simulink model "pe_pmsm_drive_code"  (R2018b)
settings: Solver=FixedStepDiscrete  StartTime=0.0  StopTime=0.5  FixedStep=2e-7  MaxStep=2.0E-6  RelTol=1e-6  AbsTol=1e-3  EnableMultiTasking=on
PreLoadFcn:
  | % Control parameters
  | Ts = 2e-6;   % Fundamental sample time
  | fsw = 2e3;   % Switching frequency (Hz)
  | fc = fsw*10; % Control loop frequency (Hz)
  | Tsc = 1/fc;  % Control loop sample time
  | 
  | % PMSM parameters
  | PM = 0.03; % Permanent magnet flux linkage
  | Ld = 2e-4;  % d-axis inductance
  | Lq = 2e-4;  % q-axis inductance
  | L0 = 2e-4;  % 0-axis inductance
  | Rs = 0.013; % Stator resistance
  | N = 6; % Number of pole pairs
  | J = 0.2; % Moment of inertia
  | 
  | % Operating and derived limits
  | Imax = 100;  % Max stator current (peak value)
  | Tmax = 1.5*N*PM*Imax; % Max lectromagnetic torque
  | fnom = 100;  % Nominal frequency (Hz)
  | rpm_nom = 60*fnom/N;      % Nominal rotor speed (rpm)
  | omegam_nom = 2*pi*fnom/N; % Nominal mechanical rotor speed
  | Pmax = omegam_nom*Tmax;     % Maximum power
values from neighbouring files (symbols this model uses):
  faero = 0.5*cd*frontarea*airdens.*speed.^2    [PMSM_code.m]
  speed = linspace(0, 60, 1000)    [PMSM_code.m]
  wheelrad = 0.3    [PMSM_code.m]
undefined symbols (not defined in the file or in its folder): DiscIntNeverNeededParam, gcbh, pe_sli_rtmsupport
libraries: nesl_utility x12, pe_lib x10, fl_lib x8, peTransforms x2, pePmsmCurrentController x1, simulink x1, peVelocityController x1
(part 2 of 2)

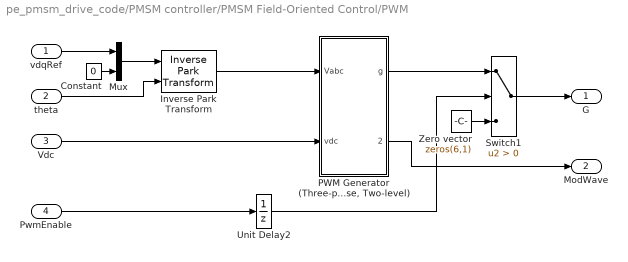
== system pe_pmsm_drive_code/PMSM controller/PMSM Field-Oriented Control/PWM ==
  vdqRef : Inport
  theta : Inport  Port=2
  Vdc : Inport  Port=3
  PwmEnable : Inport  Port=4
  Constant : Constant  Value=0  SampleTime=Tsc
  Inverse Park Transform : peTransforms/Inverse Park Transform  AxisAlignment=Q-axis  PowerInvariant=off
  Mux : Mux  Inputs=2
  "PWM Generator (Three-phase, Two-level)" : Subsystem  AncestorBlock=|  LoadFcn=pe_sli_rtmsupport( 'loadfcn', gcbh );  mask(PWM Generator (three-phase, two-level)){PWMMode=Continuous PWM (CPWM), CPWMMode=SPWM: sinusoidal PWM, DPWMMode=60 DPWM: 60 degree discontinuous PWM, SamplingMode=Natural, fsw=fsw, Ts=Ts}
      | pePwmGeneratorTwoLevel/PWM Generator
      | (Three-phase, Two-level)
      mask prompts: PWMMode "PWM mode:"; CPWMMode "Continuous PWM:"; DPWMMode "Discontinuous PWM:"; SamplingMode "Sampling mode:"; fsw "Switching frequency (Hz):"; Ts "Sample time (s):"
      mask help: This block implements a three-phase, two-level PWM waveform generator.
      mask init:
      | Tsw = 1/fsw;
      | 
      | if fsw <= 0
      |     error(message('physmod:simscape:compiler:patterns:checks:GreaterThanZero','Switching frequency'));
      | end
      | 
      | if Ts <= 0
      |     error(message('physmod:simscape:compiler:patterns:checks:GreaterThanZero','Sample time'));
      | end
      | 
      | if Ts > 1/(10*fsw)
      |     error(message('physmod:simscape:compiler:patterns:checks:LessThanOrEqual','Sample time','inverse of 10 times Switching frequency'));
      | end
      | 
      | switch SamplingMode
      |     case 'Natural'
      |         RateTransitionOnInput = -1;
      |         GateGeneratorX0 = 0;
      |     case 'Asymmetric'
      |         RateTransitionOnInput = 0.5*Tsw;
      |         GateGeneratorX0 = 0.5/fsw;
      |     case 'Symmetric'
      |         RateTransitionOnInput = Tsw;
      |         GateGeneratorX0 = 0;
      | end
      | 
      | 
      | switch PWMMode
      |     case 'Continuous PWM (CPWM)'
      |         switch CPWMMode
      |             case 'SPWM: sinusoidal PWM'
      |                 PWM = 1;
      |             case 'SVM: space vector modulation'
      |                 PWM = 2;
      |         end
      |     case 'Discontinuous PWM (DPWM)'
      |         switch DPWMMode
      |             case '60 DPWM: 60 degree discontinuous PWM'
      |                 PWM = 3;
      |             case '60 DPWM (+30 degree shift): +30 degree shift from 60 DPWM'
      |                 PWM = 4;
      |             case '60 DPWM (-30 degree shift): -30 degree shift from 60 DPWM'
      |                 PWM = 5;
      |             case '30 DPWM: 30 degree discontinuous PWM'
      |                 PWM = 6;
      |             case '120 DPWM: positive dc component'
      |                 PWM = 7;
      |             case '120 DPWM: negative dc component'
      |                 PWM = 8;
      |         end
      | end
      settings: CopyFcn=pe_sli_rtmsupport( 'copyfcn', gcbh );  DeleteFcn=pe_sli_rtmsupport( 'deletefcn', gcbh );  ModelCloseFcn=pe_sli_rtmsupport( 'modelclosefcn', gcbh );  PreSaveFcn=%pe_sli_rtmsupport( 'presavefcn', gcbh );  PostSaveFcn=pe_sli_rtmsupport( 'postsavefcn', gcbh );  PreCopyFcn=pe_sli_rtmsupport( 'precopyfcn', gcbh );  OpenFcn=pe_sli_rtmsupport( 'openfcn', gcbh );  CloseFcn=pe_sli_rtmsupport( 'closefcn', gcbh );  PreDeleteFcn=pe_sli_rtmsupport( 'predeletefcn', gcbh );
      mask Help: web(nesl_help(gcbh))
      mask TypeOptions PWMMode: Continuous PWM (CPWM) | Discontinuous PWM (DPWM)
      mask Callback PWMMode:
      | switch get_param(gcb,'PWMMode')
      |     case 'Continuous PWM (CPWM)'
      |         set_param(gcb,'MaskVisibilities',{'on';'on';'off';'on';'on';'on'})
      |     case 'Discontinuous PWM (DPWM)'
      |         set_param(gcb,'MaskVisibilities',{'on';'off';'on';'on';'on';'on'})
      | end
      mask TypeOptions CPWMMode: SPWM: sinusoidal PWM | SVM: space vector modulation
      mask TypeOptions DPWMMode: 60 DPWM: 60 degree discontinuous PWM | 60 DPWM (+30 degree shift): +30 degree shift from 60 DPWM | 60 DPWM (-30 degree shift): -30 degree shift from 60 DPWM | 30 DPWM: 30 degree discontinuous PWM | 120 DPWM: positive dc component | 120 DPWM: negative dc component
      mask TypeOptions SamplingMode: Natural | Asymmetric | Symmetric
  Switch1 : Switch  Criteria=u2 > Threshold
  Unit Delay2 : UnitDelay  SampleTime=Tsc
  Zero vector : Constant  Value=zeros(6,1)  SampleTime=Ts
  G : Outport
  ModWave : Outport  Port=2  SampleTime=Tsc
  wires:
  Unit Delay2/1 -> Switch1/2
  Vdc/1 -> "PWM Generator (Three-phase, Two-level)"/2(vdc)
  Inverse Park Transform/1 -> "PWM Generator (Three-phase, Two-level)"/1(Vabc)
  Switch1/1 -> G/1
  Zero vector/1 -> Switch1/3
  PwmEnable/1 -> Unit Delay2/1
  "PWM Generator (Three-phase, Two-level)"/1(g) -> Switch1/1
  "PWM Generator (Three-phase, Two-level)"/2(ModWave) -> ModWave/1
  Constant/1 -> Mux/2
  Mux/1 -> Inverse Park Transform/1
  vdqRef/1 -> Mux/1
  theta/1 -> Inverse Park Transform/2

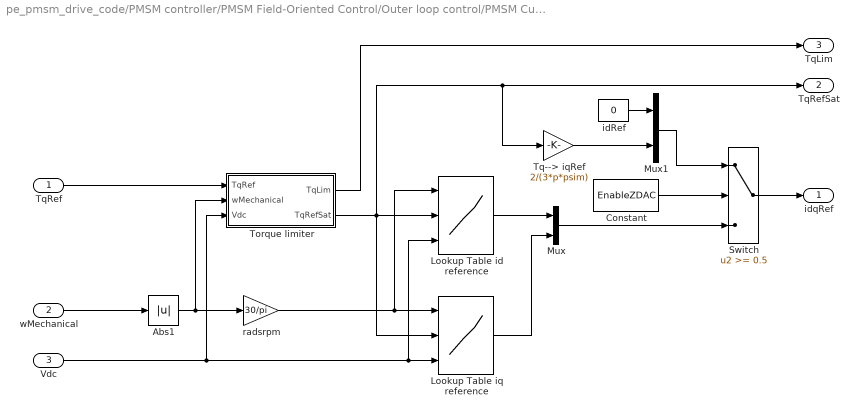
== system pe_pmsm_drive_code/PMSM controller/PMSM Field-Oriented Control/Outer loop control/PMSM Current Reference Generator ==
  TqRef : Inport  SampleTime=Ts
  wMechanical : Inport  Port=2  SampleTime=Ts
  Vdc : Inport  Port=3  SampleTime=Ts
  Abs1 : Abs
  Constant : Constant  Value=EnableZDAC  SampleTime=Ts
  Lookup Table id reference : Lookup_n-D  NumberOfTableDimensions=3  BreakpointsForDimension1=rpmVec  BreakpointsForDimension2=TqVec  BreakpointsForDimension3=VdcVec  Table=idMatrix  RemoveProtectionInput=on  InputSameDT=on
  Lookup Table iq reference : Lookup_n-D  NumberOfTableDimensions=3  BreakpointsForDimension1=rpmVec  BreakpointsForDimension2=TqVec  BreakpointsForDimension3=VdcVec  Table=iqMatrix  RemoveProtectionInput=on  MaximumIndicesForEachDimension=[1, 2, 1]  InputSameDT=on
  Mux : Mux  Inputs=2
  Mux1 : Mux  Inputs=2
  Switch : Switch  Threshold=0.5
  Torque limiter : Subsystem
  Tq--> iqRef : Gain  Gain=2/(3*p*psim)
  idRef : Constant  Value=0  SampleTime=Ts
  radsrpm : Gain  Gain=30/pi
  idqRef : Outport
  TqRefSat : Outport  Port=2
  TqLim : Outport  Port=3
  wires:
  Lookup Table id reference/1 -> Mux/1
  Lookup Table iq reference/1 -> Mux/2
  Torque limiter/2(TqRefSat) -> Lookup Table iq reference/2, TqRefSat/1, Tq--> iqRef/1, Lookup Table id reference/2
  Torque limiter/1(TqLim) -> TqLim/1
  radsrpm/1 -> Lookup Table id reference/1, Lookup Table iq reference/1
  Abs1/1 -> Torque limiter/2(wMechanical), radsrpm/1
  Mux1/1 -> Switch/1
  Mux/1 -> Switch/3
  Switch/1 -> idqRef/1
  idRef/1 -> Mux1/1
  Tq--> iqRef/1 -> Mux1/2
  TqRef/1 -> Torque limiter/1(TqRef)
  wMechanical/1 -> Abs1/1
  Vdc/1 -> Lookup Table id reference/3, Lookup Table iq reference/3, Torque limiter/3(Vdc)
  Constant/1 -> Switch/2

== system pe_pmsm_drive_code/PMSM controller/PMSM Field-Oriented Control/Outer loop control/Tq Selector ==
  Reference : Inport
  TqRefUnsat : Inport  Port=2
  Constant : Constant  Value=CtrlMode  SampleTime=Tsc
  Switch : Switch  Criteria=u2 > Threshold  Threshold=1.5
  TqRef : Outport
  wires:
  Switch/1 -> TqRef/1
  Constant/1 -> Switch/2
  TqRefUnsat/1 -> Switch/3
  Reference/1 -> Switch/1

== system pe_pmsm_drive_code/PMSM controller/PMSM Field-Oriented Control/PWM/PWM Generator (Three-phase, Two-level) ==
  Vabc : Inport
  vdc : Inport  Port=2
  Data Type Conversion : DataTypeConversion
  Data Type Conversion1 : DataTypeConversion
  Gate Signal Generator : Subsystem
  Rate Transition : RateTransition  Deterministic=off
  Rate Transition1 : RateTransition  Deterministic=off
  Switching Time Calculation : MATLAB Function  TreatAsAtomicUnit=on
  avoid division by 0 : Saturate  UpperLimit=inf  LowerLimit=eps
  g : Outport
  ModWave : Outport  Port=2
  wires:
  Vabc/1 -> Rate Transition/1
  Switching Time Calculation/1(TgabcON) -> Gate Signal Generator/1(TgabcON)
  Switching Time Calculation/2(TgabcOFF) -> Gate Signal Generator/2(TgabcOFF)
  Gate Signal Generator/1(s) -> Data Type Conversion/1
  Data Type Conversion/1 -> g/1
  Switching Time Calculation/3(ModWave) -> Data Type Conversion1/1
  Rate Transition/1 -> Switching Time Calculation/1(Vabc)
  avoid division by 0/1 -> Switching Time Calculation/2(vdc)
  Data Type Conversion1/1 -> ModWave/1
  vdc/1 -> Rate Transition1/1
  Rate Transition1/1 -> avoid division by 0/1

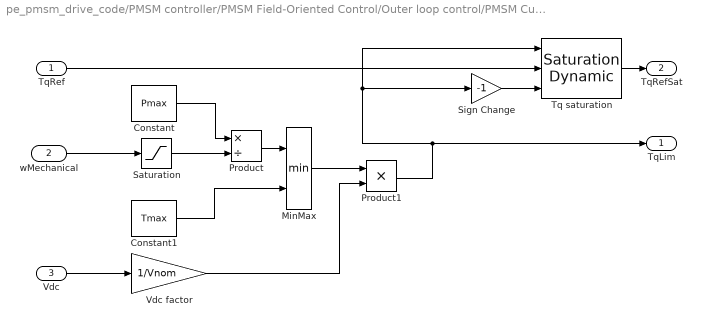
== system pe_pmsm_drive_code/PMSM controller/PMSM Field-Oriented Control/Outer loop control/PMSM Current Reference Generator/Torque limiter ==
  TqRef : Inport
  wMechanical : Inport  Port=2
  Vdc : Inport  Port=3
  Constant : Constant  Value=Pmax  SampleTime=Ts
  Constant1 : Constant  Value=Tmax  SampleTime=Ts
  MinMax : MinMax  Inputs=2
  Product : Product  Inputs=*/
  Product1 : Product
  Saturation : Saturate  UpperLimit=inf  LowerLimit=Pmax/Tmax
  Sign Change : Gain  Gain=-1
  Tq saturation : simulink/Discontinuities/Saturation Dynamic  OutMin=[]  OutMax=[]  OutDataTypeStr=Inherit: Same as second input  OutDataType=fixdt(1, 16)  OutScaling=2^-10  DoSatur=off
  Vdc factor : Gain  Gain=1/Vnom
  TqLim : Outport
  TqRefSat : Outport  Port=2
  wires:
  Tq saturation/1 -> TqRefSat/1
  Vdc/1 -> Vdc factor/1
  Constant1/1 -> MinMax/2
  wMechanical/1 -> Saturation/1
  Product/1 -> MinMax/1
  Constant/1 -> Product/1
  Saturation/1 -> Product/2
  Sign Change/1 -> Tq saturation/3
  MinMax/1 -> Product1/1
  Vdc factor/1 -> Product1/2
  TqRef/1 -> Tq saturation/2
  Product1/1 -> Sign Change/1, Tq saturation/1, TqLim/1

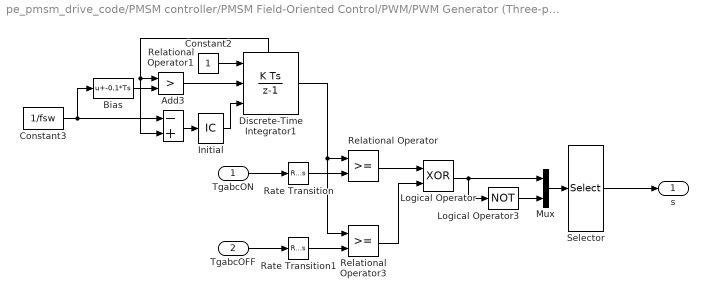
== system pe_pmsm_drive_code/PMSM controller/PMSM Field-Oriented Control/PWM/PWM Generator (Three-phase, Two-level)/Gate Signal Generator ==
  TgabcON : Inport
  TgabcOFF : Inport  Port=2
  Add3 : Sum  Inputs=-+
  Bias : Bias  Bias=-0.1*Ts
  Constant2 : Constant
  Constant3 : Constant  Value=1/fsw
  Discrete-Time Integrator1 : DiscreteIntegrator  ExternalReset=rising  InitialConditionSource=external  SampleTime=Ts  ShowStatePort=on  ICPrevOutput=DiscIntNeverNeededParam  ICPrevScaledInput=DiscIntNeverNeededParam
  Initial : InitialCondition  Value=GateGeneratorX0
  Logical Operator : Logic  Operator=XOR  AllPortsSameDT=off  OutDataTypeStr=boolean
  Logical Operator3 : Logic  Operator=NOT  AllPortsSameDT=off  OutDataTypeStr=boolean
  Mux : Mux  Inputs=2
  Rate Transition : RateTransition  Deterministic=off
  Rate Transition1 : RateTransition  Deterministic=off
  Relational Operator : RelationalOperator  OutDataTypeStr=boolean  RndMeth=Nearest
  Relational Operator1 : RelationalOperator  Operator=>  OutDataTypeStr=boolean  RndMeth=Nearest
  Relational Operator3 : RelationalOperator  OutDataTypeStr=boolean  RndMeth=Nearest
  Selector : Selector  InputPortWidth=6  IndexOptions=Index vector (dialog)  Indices=[1 4 2 5 3 6]  OutputSizes=1
  s : Outport
  wires:
  Relational Operator3/1 -> Logical Operator/2
  Relational Operator/1 -> Logical Operator/1
  Logical Operator/1 -> Logical Operator3/1, Mux/1
  Logical Operator3/1 -> Mux/2
  Mux/1 -> Selector/1
  Selector/1 -> s/1
  Discrete-Time Integrator1/1 -> Relational Operator3/1, Relational Operator/1
  Bias/1 -> Relational Operator1/2
  Relational Operator1/1 -> Discrete-Time Integrator1/2
  Add3/1 -> Initial/1
  Initial/1 -> Discrete-Time Integrator1/3
  Constant2/1 -> Discrete-Time Integrator1/1
  Discrete-Time Integrator1/State -> Add3/2, Relational Operator1/1
  Constant3/1 -> Bias/1, Add3/1
  TgabcON/1 -> Rate Transition/1
  Rate Transition/1 -> Relational Operator/2
  TgabcOFF/1 -> Rate Transition1/1
  Rate Transition1/1 -> Relational Operator3/2

== matlab function pe_pmsm_drive_code/PMSM controller/PMSM Field-Oriented Control/PWM/PWM Generator (Three-phase, Two-level)/Switching Time Calculation ==
  settings: sampleTime=1
  data: Vabc input; TgabcON output; vdc input; TgabcOFF output; ModWave output; fsw parameter; PWM parameter
function [TgabcON,TgabcOFF,ModWave]  = switchingTime(Vabc,vdc,fsw,PWM)

[TgabcON,TgabcOFF,ModWave] = pe.control.pwmSwitchingTimeTwoLevel(Vabc,vdc,fsw,PWM);
